simulink library "robolocks"  (Simulink 7.6)
settings: Solver=ode45  StartTime=0.0  StopTime=10.0  RelTol=1e-3
values from neighbouring files (symbols this model uses):
  q = 1    [quadrotor_plot.m]
  z = x(1:3)    [nrotor_dynamics.m]    (also in quadrotor_dynamics.m; quadrotor_plot.m = [u(1);u(2);u(3)])
undefined symbols (not defined in the file or in its folder): angdiff, Bicycle, cam, camera, camera2, Circle, cond, delta2tr, Dynamics, eul2T, eul2tr, fkine, ijacob, Inverse, invJac, jacob0, jacobn, jtraj, lspb, numcols, pinvJac, Plot, points, qd, qdd, Quadcopter, RNE, rne, roblocks_old, robot, Robot, rpy2T, rpy2tr, T2eul, T2rpy, T2xyz, test, tr2delta, tr2diff, tr2eul, tr2rpy, transl, trnorm, trotx, xyz2T
settings Model: Creator=n6334687  LastModifiedBy=n6334687

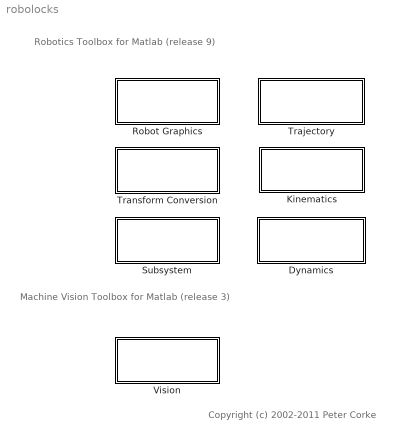
== system robolocks ==
  note: Robotics Toolbox for Matlab
      | (release 9)
  note: Machine Vision Toolbox for Matlab
      | (release 3)
  note: Copyright (c) 2002-2011 Peter Corke
  Dynamics : Subsystem
      mask Display:
      | color('darkBlue')
      | disp('Dynamics')
  Kinematics : Subsystem  AncestorBlock=test/Dynamics
      mask Display:
      | color('darkBlue')
      | disp('Kinematics')
  Robot Graphics : Subsystem  AncestorBlock=test/Plot
      mask Display:
      | color('darkBlue')
      | disp('Robot Graphics')
  Subsystem : Subsystem
      mask Display:
      | color('darkBlue')
      | disp('Transform')
  "Trajectory " : Subsystem
      mask Display:
      | color('darkBlue')
      | disp('Trajectory')
  Transform Conversion : Subsystem
      mask Display:
      | color('darkBlue')
      | disp('Transform Conversion')
  Vision : Subsystem
      mask Display:
      | color('Black')
      | disp('Vision')

== system robolocks/Dynamics ==
  note: Dynamics
  note: Arm-type robot
  note: Quadcopter
  note: Mobile robot
  Bicycle : Subsystem  AncestorBlock=roblocks_old/Bicycle  mask{accel=1, vlim=1, alim=2, x0=[0, 0, 0], handbrake=0}
      mask prompts: accel "Acceleration"; vlim "Velocity limit"; alim "Steering limits"; x0 "Initial state (x, y, theta)"
  Control Mixer : Subsystem  AncestorBlock=roblocks_old/Control Mixer
  Quadcopter : Subsystem  AncestorBlock=roblocks_old/Quadcopter  mask{quad=0}
      mask prompts: quad "Quadcopter params"
  RNE : Subsystem  AncestorBlock=roblocks_old/RNE  mask{robot=robot, grav=[0 0 9.81]}
      mask prompts: robot "Robot object"; grav "Gravity"
      mask help: Rigid-body inverse dynamics.
      mask init:
      | if isa(robot, 'SerialLink')
      |     n = robot.n
      |     rname = robot.name;
      | else
      |     n = 0;
      |     rname = '';
      | end
      mask Help: Given a robot dynamic model and joint angle, rate and acceleration determine the required joint torque.  Useful for computed and inverse torque control schemes.
      mask Display:
      | port_label('output', 1, 'Q')
      | port_label('input', 1, 'q')
      | port_label('input', 2, 'qd')
      | port_label('input', 3, 'qdd')
      | text(0.9, 0.9,  rname, 'horizontalAlignment', 'right')
  Robot : Subsystem  AncestorBlock=roblocks_old/Robot  mask{robot=robot, q0=[0 0 0 0 0 0]}
      mask prompts: robot "Robot object"; q0 "Initial state"
      mask help: Rigid-body dynamic model of robot.
      mask init:
      | if isa(robot, 'SerialLink')
      |     rname = robot.name;
      |     fprintf('**robot name is %s\n', rname);
      | else
      |     rname = '';
      |     n = 0
      | end
      mask Help: Simulates the forward (direct) rigid-body dynamics of the robot described by the given robot object.
      mask Display:
      | port_label('input', 1, 'Q')
      | port_label('output', 1, 'q')
      | port_label('output', 2, 'qd')
      | port_label('output', 3, 'qdd')
      | text(0.1, 0.9,  rname, 'horizontalAlignment', 'left')
  wires:
  ? -> RNE/2(qd)

== system robolocks/Kinematics ==
  note: Kinematics
  fkine : Subsystem  AncestorBlock=roblocks_old/fkine  mask{robot=robot}
      mask prompts: robot "Robot object"
      mask help: Robot forward kinematics.
      mask Help: Compute homogeneous transform for robot end-effector given joint angles.
      mask Display:
      | port_label('input', 1, 'q')
      | port_label('output', 1, 'T')
      | text(0.9, 0.9, robot.name,  'horizontalAlignment', 'right')
  ijacob : Subsystem  AncestorBlock=roblocks_old/ijacob
      mask Description:
      | Robot inverse Jacobian for world coordinates.
      | 
      | Only valid for square jacobians (ie/ 6DOF robots)
      mask Display:
      | text(0.4, 0.7, 'J', 'verticalAlignment', 'top', 'horizontalAlignment', 'left')
      | text(0.65, 0.65, '-1', 'verticalAlignment', 'bottom', 'horizontalAlignment', 'right')
      | port_label('input', 1, 'J');
      | port_label('output', 1, 'Ji')
  "jacob0 " : Subsystem  AncestorBlock=roblocks_old/jacob0  mask{robot=robot}
      mask prompts: robot "Robot object"
      mask help: Robot Jacobian for end-effector coordinates
      mask init:
      | n=robot.n;
      mask Display:
      | text(0.4, 0.7, 'J', 'verticalAlignment', 'top', 'horizontalAlignment', 'left')
      | text(0.4, 0.7, '0', 'verticalAlignment', 'bottom', 'horizontalAlignment', 'right')
      | text(0.5, 0.2, robot.name,  'horizontalAlignment', 'center')
      | port_label('input', 1, 'q')
      | port_label('output', 1, 'J')
  jacobn : Subsystem  AncestorBlock=roblocks_old/jacobn  mask{robot=robot}
      mask prompts: robot "Robot object"
      mask help: Robot Jacobian for end-effector coordinates
      mask init:
      | n=robot.n;
      mask Display:
      | text(0.5, 0.4, 'J', 'verticalAlignment', 'top', 'horizontalAlignment', 'left')
      | text(0.5, 0.4, 'n', 'verticalAlignment', 'bottom', 'horizontalAlignment', 'right')
      | text(0.9, 0.9, robot.name,  'horizontalAlignment', 'right')
      | port_label('input', 1, 'q')
      | port_label('output', 1, 'J')
  tr2diff : Subsystem  AncestorBlock=roblocks_old/tr2diff  mask{robot=robot}
      mask prompts: robot "Robot object"
      mask help: Robot forward kinematics.
      mask Help: Compute homogeneous transform for robot end-effector given joint angles.
      mask Display:
      | port_label('input', 1, 'T1')
      | port_label('input', 2, 'T2')
      | port_label('output', 1, 'dx')

== system robolocks/Robot Graphics ==
  note: Robot
      | Graphics
  Quadcopter plot : Subsystem  AncestorBlock=roblocks_old/Quadcopter plot
  plot : Subsystem  AncestorBlock=roblocks_old/plot  mask{robot=robot}
      mask prompts: robot "Name of robot"
      mask help: Graphical robot display.
      mask init:
      | if isa(robot, 'SerialLink')
      |     plot(robot,zeros(1,robot.n));
      | rname = robot.name;
      | fprintf('**robot name is %s\n', rname);
      | else
      |     rname = '';
      | end
      mask Help: This block graphically displays the named robot
      mask Display:
      | text(0.5, 0.9,  rname, 'horizontalAlignment', 'center')
      | port_label('input', 1, 'q')

== system robolocks/Subsystem ==
  note: Transform
  Inverse : Subsystem  AncestorBlock=roblocks_old/Inverse
  Post multiply : Subsystem  AncestorBlock=roblocks_old/Post multiply  mask{T2=0}
      mask help: Premultiply incoming transform by a constant transformation
  Pre multiply : Subsystem  AncestorBlock=roblocks_old/Pre multiply  mask{T=0}
      mask prompts: T "T1"
      mask help: Post multiply incoming transform by constant transform.

== system robolocks/Trajectory  ==
  note: Trajectory
  Circle : Subsystem  AncestorBlock=roblocks_old/Circle  mask{radius=1, freq=0.2}
      mask prompts: freq "Frequency (rev/s)"
  angdiff : Subsystem  AncestorBlock=roblocks_old/angdiff
  jtraj : Subsystem  AncestorBlock=roblocks_old/jtraj  mask{q0=[0 0 0 0 0 0], qf=[pi/4 pi/2 -pi/2 0 0 0], tmax=10}
      mask help: Joint interpolated trajectory.
      mask init:
      | n = length(q0);
      | if length(q0) ~= length(qf) ,
      |  error('q0 and qf must be same length')
      | end
      | t=[0:100]'/100*tmax;
      | [q,qd,qdd] = jtraj(q0, qf, t);
      mask Help:
      | Generate quintic polynomial to move from initial to final joint angles as specified.  Initial and final velocity are assumed to be zero.
      | 
      | Outputs joint angles as well as joint angle rates.
      mask Display:
      | port_label('output', 1, 'q')
      | port_label('output', 2, 'qd')
      | port_label('output', 3, 'qdd')
  lspb : Subsystem  AncestorBlock=roblocks_old/lspb  mask{q0=0, qf=0, tmax=0}
      mask help: Scalar trajectory.
      mask init:
      | n = length(q0);
      | if length(q0) ~= length(qf) ,
      |  error('q0 and qf must be same length')
      | end
      | t=[0:1000]'/1000*tmax;
      | [q,qd,qdd] = lspb(q0, qf, t);
      mask Help:
      | Generate linear segment with polynomial blend to move from initial to final joint angles as specified.  Initial and final velocity are assumed to be zero.
      | 
      | Outputs joint angles as well as joint angle rates and acceleration.
  pose integral : Subsystem  AncestorBlock=roblocks_old/pose integral  mask{T0=transl(1,1,-3)*trotx(0.2), dt=0.02}
      mask prompts: T0 "Initial pose (hom transform)"; dt "Sample interval (s)"

== system robolocks/Transform Conversion ==
  note: Transform
      | conversion
  T2eul : Subsystem  AncestorBlock=roblocks_old/T2eul
      mask Description: Convert transform to Euler angles.
  T2rpy : Subsystem  AncestorBlock=roblocks_old/T2rpy
      mask Description: Convert transform to roll/pitch/yaw angles.
  T2xyz : Subsystem  AncestorBlock=roblocks_old/T2xyz
      mask Description: Convert transform to xyz scalars
  eul2T : Subsystem  AncestorBlock=roblocks_old/eul2T
      mask Description: Convert Euler angles to transform.
  rpy2T : Subsystem  AncestorBlock=roblocks_old/rpy2T
      mask Description: Convert roll/pitch/yaw angles to transform.
  xyz2T : Subsystem  AncestorBlock=roblocks_old/xyz2T
      mask Description: Convert xyz scalars to transform.

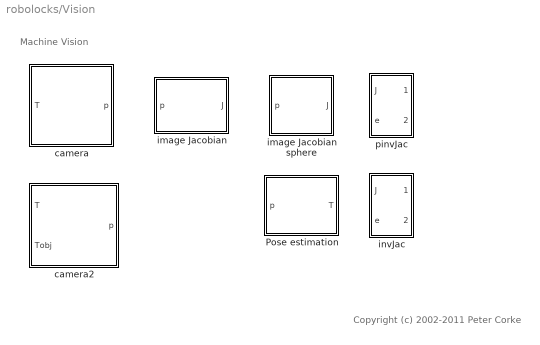
== system robolocks/Vision ==
  note: Machine Vision
  note: Copyright (c) 2002-2011 Peter Corke
  Pose estimation : Subsystem  AncestorBlock=roblocks_old/Pose estimation  mask{cam=0, P=0}
      mask prompts: cam "Camera"; P "Points (3xN)"
  camera : Subsystem  AncestorBlock=roblocks_old/camera  mask{cam=, points=}
      mask prompts: cam "Camera"; points "Points (3xN)"
  camera2 : Subsystem  AncestorBlock=roblocks_old/camera2
  image Jacobian : Subsystem  AncestorBlock=roblocks_old/image Jacobian  mask{cam=, z=}
      mask prompts: cam "Camera"; z "Assumed depth (m)"
  image Jacobian sphere : Subsystem  AncestorBlock=|
      | roblocks_old/image
      | Jacobian
      | sphere
  invJac : Subsystem  AncestorBlock=roblocks_old/invJac
  pinvJac : Subsystem  AncestorBlock=roblocks_old/pinvJac

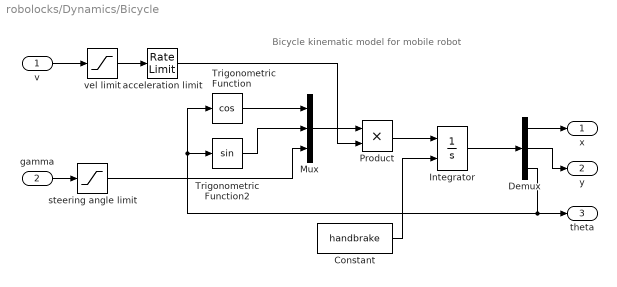
== system robolocks/Dynamics/Bicycle ==
  note: Bicycle kinematic model for mobile robot
  v : Inport
  gamma : Inport  Port=2
  Constant : Constant  Value=handbrake
  Demux : Demux  Outputs=3
  Integrator : Integrator  ExternalReset=level  InitialCondition=x0
  Mux : Mux  Inputs=3
  Product : Product  RndMeth=Zero
  Trigonometric Function : Trigonometry  Operator=cos
  Trigonometric Function2 : Trigonometry
  acceleration limit : RateLimiter  RisingSlewLimit=accel  FallingSlewLimit=-accel  SampleTimeMode=inherited
  steering angle limit : Saturate  UpperLimit=alim  LowerLimit=-alim
  vel limit : Saturate  UpperLimit=vlim  LowerLimit=-vlim
  x : Outport
  y : Outport  Port=2
  theta : Outport  Port=3
  wires:
  Constant/1 -> Integrator/2
  steering angle limit/1 -> Mux/3
  Trigonometric Function2/1 -> Mux/2
  vel limit/1 -> acceleration limit/1
  Mux/1 -> Product/1
  v/1 -> vel limit/1
  gamma/1 -> steering angle limit/1
  Demux/2 -> y/1
  Demux/1 -> x/1
  Demux/3 -> theta/1, Trigonometric Function2/1, Trigonometric Function/1
  Integrator/1 -> Demux/1
  Product/1 -> Integrator/1
  acceleration limit/1 -> Product/2
  Trigonometric Function/1 -> Mux/1

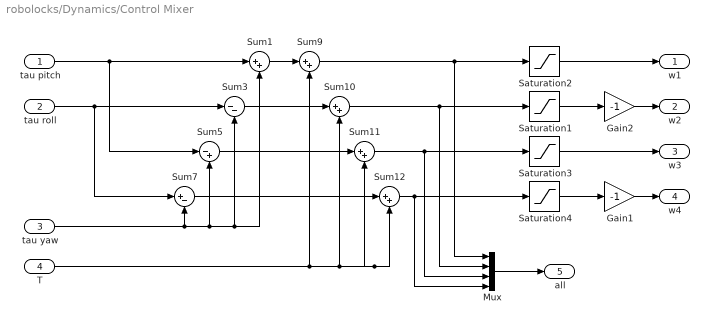
== system robolocks/Dynamics/Control Mixer ==
  tau pitch : Inport
  tau roll : Inport  Port=2
  tau yaw : Inport  Port=3
  T : Inport  Port=4
  Gain1 : Gain  Gain=-1
  Gain2 : Gain  Gain=-1
  Mux : Mux
  Saturation{1..4} (4 alike) : Saturate  UpperLimit=1000  LowerLimit=700
  Sum{1,9..12} (5 alike) : Sum  Inputs=|++  SaturateOnIntegerOverflow=on  InputSameDT=on  OutDataTypeStr=Inherit: Same as first input
  Sum3 : Sum  Inputs=|--  SaturateOnIntegerOverflow=on  InputSameDT=on  OutDataTypeStr=Inherit: Same as first input
  Sum5 : Sum  Inputs=|-+  SaturateOnIntegerOverflow=on  InputSameDT=on  OutDataTypeStr=Inherit: Same as first input
  Sum7 : Sum  Inputs=|+-  SaturateOnIntegerOverflow=on  InputSameDT=on  OutDataTypeStr=Inherit: Same as first input
  w1 : Outport
  w2 : Outport  Port=2
  w3 : Outport  Port=3
  w4 : Outport  Port=4
  all : Outport  Port=5
  wires:
  Gain1/1 -> w4/1
  Gain2/1 -> w2/1
  Mux/1 -> all/1
  tau roll/1 -> Sum7/1, Sum3/1
  T/1 -> Sum9/2, Sum10/2, Sum11/2, Sum12/2
  Sum12/1 -> Mux/4, Saturation4/1
  Sum11/1 -> Mux/3, Saturation3/1
  Sum10/1 -> Mux/2, Saturation1/1
  Sum9/1 -> Mux/1, Saturation2/1
  Sum7/1 -> Sum12/1
  Sum5/1 -> Sum11/1
  Sum3/1 -> Sum10/1
  Sum1/1 -> Sum9/1
  tau pitch/1 -> Sum5/1, Sum1/1
  Saturation4/1 -> Gain1/1
  Saturation3/1 -> w3/1
  Saturation1/1 -> Gain2/1
  Saturation2/1 -> w1/1
  tau yaw/1 -> Sum1/2, Sum3/2, Sum5/2, Sum7/2

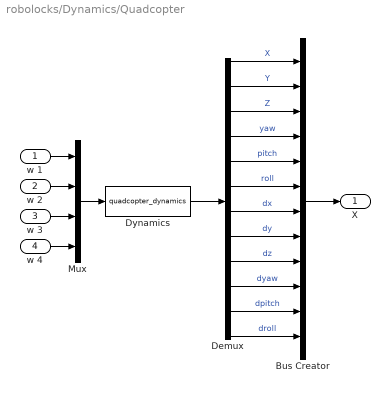
== system robolocks/Dynamics/Quadcopter ==
  w 1 : Inport
  w 2 : Inport  Port=2
  w 3 : Inport  Port=3
  w 4 : Inport  Port=4
  Bus Creator : BusCreator  Inputs='X','Y','Z','yaw','pitch','roll','dx','dy','dz','dyaw','dpitch','droll'
  Demux : Demux  Outputs=12
  Dynamics : S-Function  FunctionName=quadcopter_dynamics  Parameters=quad  EnableBusSupport=off
  Mux : Mux
  X : Outport
  wires:
  Demux/12 -> Bus Creator/12  "droll"
  Demux/11 -> Bus Creator/11  "dpitch"
  Demux/10 -> Bus Creator/10  "dyaw"
  Dynamics/1 -> Demux/1
  Bus Creator/1 -> X/1
  Demux/8 -> Bus Creator/8  "dy"
  Demux/6 -> Bus Creator/6  "roll"
  Demux/2 -> Bus Creator/2  "Y"
  Demux/9 -> Bus Creator/9  "dz"
  Demux/7 -> Bus Creator/7  "dx"
  w 4/1 -> Mux/4
  w 3/1 -> Mux/3
  w 2/1 -> Mux/2
  w 1/1 -> Mux/1
  Demux/5 -> Bus Creator/5  "pitch"
  Demux/4 -> Bus Creator/4  "yaw"
  Demux/3 -> Bus Creator/3  "Z"
  Demux/1 -> Bus Creator/1  "X"
  Mux/1 -> Dynamics/1

== system robolocks/Dynamics/RNE ==
  q : Inport
  qd : Inport  Port=2
  qdd : Inport  Port=3
  MATLAB Fcn : MATLABFcn  MATLABFcn=rne(robot, u(1:n)', u(n+1:2*n)', u(2*n+1:3*n)')  OutputDimensions=n
  Mux : Mux  Inputs=3
  Q : Outport
  wires:
  Mux/1 -> MATLAB Fcn/1
  q/1 -> Mux/1
  qd/1 -> Mux/2
  qdd/1 -> Mux/3
  MATLAB Fcn/1 -> Q/1

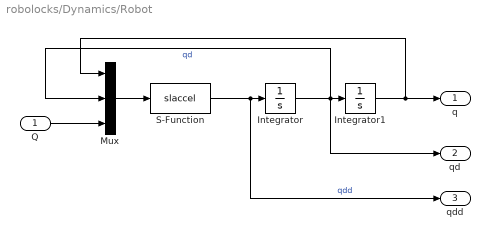
== system robolocks/Dynamics/Robot ==
  Q : Inport
  Integrator : Integrator
  Integrator1 : Integrator
  Mux : Mux  Inputs=3
  S-Function : S-Function  FunctionName=slaccel  Parameters=robot  EnableBusSupport=off
  q : Outport
  qd : Outport  Port=2
  qdd : Outport  Port=3
  wires:
  Integrator1/1 -> Mux/1, q/1
  Q/1 -> Mux/3
  Integrator/1 -> Mux/2, Integrator1/1, qd/1  "qd"
  Mux/1 -> S-Function/1
  S-Function/1 -> Integrator/1, qdd/1  "qdd"

== system robolocks/Kinematics/fkine ==
  q : Inport
  MATLAB Fcn : MATLABFcn  MATLABFcn=fkine(robot,u)  OutputDimensions=[4 4]  Output1D=off
  T : Outport
  wires:
  MATLAB Fcn/1 -> T/1
  q/1 -> MATLAB Fcn/1

== system robolocks/Kinematics/ijacob ==
  J : Inport
  inverse jacobian : MATLABFcn  MATLABFcn=inv(u)  Output1D=off
  Ji : Outport
  wires:
  J/1 -> inverse jacobian/1
  inverse jacobian/1 -> Ji/1

== system robolocks/Kinematics/jacob0  ==
  q : Inport
  MATLAB Fcn : MATLABFcn  MATLABFcn=jacob0(robot,u)  OutputDimensions=[6 n]  Output1D=off
  J : Outport
  wires:
  q/1 -> MATLAB Fcn/1
  MATLAB Fcn/1 -> J/1

== system robolocks/Kinematics/jacobn ==
  q : Inport
  MATLAB Fcn : MATLABFcn  MATLABFcn=jacobn(robot,u)  OutputDimensions=[6 n]  Output1D=off
  J : Outport
  wires:
  q/1 -> MATLAB Fcn/1
  MATLAB Fcn/1 -> J/1

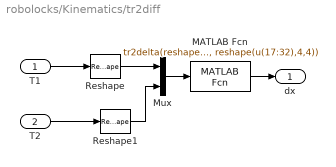
== system robolocks/Kinematics/tr2diff ==
  T1 : Inport
  T2 : Inport  Port=2
  MATLAB Fcn : MATLABFcn  MATLABFcn=tr2delta(reshape(u(1:16),4,4), reshape(u(17:32),4,4))  OutputDimensions=6
  Mux : Mux  Inputs=2
  Reshape : Reshape
  Reshape1 : Reshape
  dx : Outport
  wires:
  Reshape1/1 -> Mux/2
  Reshape/1 -> Mux/1
  Mux/1 -> MATLAB Fcn/1
  T2/1 -> Reshape1/1
  T1/1 -> Reshape/1
  MATLAB Fcn/1 -> dx/1

== system robolocks/Robot Graphics/Quadcopter plot ==
  X : Inport
  Bus Selector1 : BusSelector  OutputSignals=X,Y,Z,yaw,pitch,roll  OutputAsBus=on
  Plotter : S-Function  FunctionName=quadcopter_plot  Parameters=[2,10], 1, 1  EnableBusSupport=off
  wires:
  Bus Selector1/1 -> Plotter/1
  X/1 -> Bus Selector1/1

== system robolocks/Robot Graphics/plot ==
  q : Inport
  S-Function : S-Function  FunctionName=slplotbot  Parameters=robot  EnableBusSupport=off
  wires:
  q/1 -> S-Function/1

== system robolocks/Subsystem/Inverse ==
  T : Inport
  MATLAB Fcn : MATLABFcn  MATLABFcn=inv(u)  OutputDimensions=[4,4]  Output1D=off
  invT : Outport
  wires:
  MATLAB Fcn/1 -> invT/1
  T/1 -> MATLAB Fcn/1

== system robolocks/Subsystem/Post multiply ==
  T1 : Inport
  Constant : Constant  Value=T2
  Product : Product  Multiplication=Matrix(*)  RndMeth=Zero
  T : Outport
  wires:
  T1/1 -> Product/1
  Constant/1 -> Product/2
  Product/1 -> T/1

== system robolocks/Subsystem/Pre multiply ==
  T2 : Inport
  Constant : Constant  Value=T  VectorParams1D=off
  Product : Product  Multiplication=Matrix(*)  RndMeth=Zero
  T : Outport
  wires:
  T2/1 -> Product/2
  Product/1 -> T/1
  Constant/1 -> Product/1

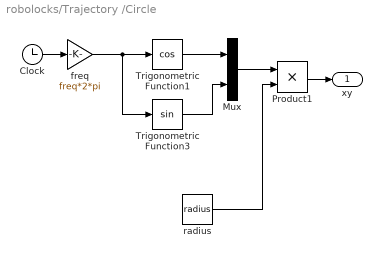
== system robolocks/Trajectory /Circle ==
  Clock : Clock
      settings: Decimation=10
  Mux : Mux  Inputs=2
  Product1 : Product  RndMeth=Zero
  Trigonometric Function1 : Trigonometry  Operator=cos
  Trigonometric Function3 : Trigonometry
  freq : Gain  Gain=freq*2*pi
  radius : Constant  Value=radius
  xy : Outport
  wires:
  Trigonometric Function3/1 -> Mux/2
  Trigonometric Function1/1 -> Mux/1
  Mux/1 -> Product1/1
  radius/1 -> Product1/2
  Clock/1 -> freq/1
  Product1/1 -> xy/1
  freq/1 -> Trigonometric Function1/1, Trigonometric Function3/1

== system robolocks/Trajectory /angdiff ==
  + : Inport
  - : Inport  Port=2
  MATLAB Fcn : MATLABFcn  MATLABFcn=angdiff(u(1), u(2))
  Mux : Mux  Inputs=2
  d : Outport
  wires:
  -/1 -> Mux/2
  MATLAB Fcn/1 -> d/1
  Mux/1 -> MATLAB Fcn/1
  +/1 -> Mux/1

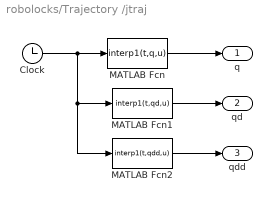
== system robolocks/Trajectory /jtraj ==
  Clock : Clock
      settings: Decimation=10
  MATLAB Fcn : MATLABFcn  MATLABFcn=interp1(t,q,u)  OutputDimensions=n
  MATLAB Fcn1 : MATLABFcn  MATLABFcn=interp1(t,qd,u)  OutputDimensions=n
  MATLAB Fcn2 : MATLABFcn  MATLABFcn=interp1(t,qdd,u)  OutputDimensions=n
  q : Outport
  qd : Outport  Port=2
  qdd : Outport  Port=3
  wires:
  MATLAB Fcn2/1 -> qdd/1
  Clock/1 -> MATLAB Fcn2/1, MATLAB Fcn1/1, MATLAB Fcn/1
  MATLAB Fcn1/1 -> qd/1
  MATLAB Fcn/1 -> q/1

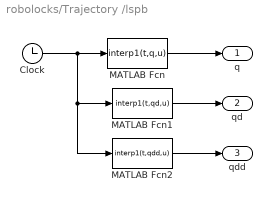
== system robolocks/Trajectory /lspb ==
  Clock : Clock
      settings: Decimation=10
  MATLAB Fcn : MATLABFcn  MATLABFcn=interp1(t,q,u)  OutputDimensions=n
  MATLAB Fcn1 : MATLABFcn  MATLABFcn=interp1(t,qd,u)  OutputDimensions=n
  MATLAB Fcn2 : MATLABFcn  MATLABFcn=interp1(t,qdd,u)  OutputDimensions=n
  q : Outport
  qd : Outport  Port=2
  qdd : Outport  Port=3
  wires:
  MATLAB Fcn/1 -> q/1
  MATLAB Fcn1/1 -> qd/1
  Clock/1 -> MATLAB Fcn/1, MATLAB Fcn1/1, MATLAB Fcn2/1
  MATLAB Fcn2/1 -> qdd/1

== system robolocks/Trajectory /pose integral ==
  v : Inport
  MATLAB Fcn3 : MATLABFcn  MATLABFcn=delta2tr(u)  Output1D=off
  Product : Product  Multiplication=Matrix(*)  RndMeth=Zero
  Unit Delay : UnitDelay  X0=T0  SampleTime=dt
  trnorm : MATLABFcn  MATLABFcn=trnorm(u)  Output1D=off
  T : Outport
  wires:
  v/1 -> MATLAB Fcn3/1
  trnorm/1 -> Unit Delay/1
  MATLAB Fcn3/1 -> Product/1
  Unit Delay/1 -> T/1, Product/2
  Product/1 -> trnorm/1

== system robolocks/Transform Conversion/T2eul ==
  T : Inport
  Demux : Demux  Outputs=3
  MATLAB Fcn : MATLABFcn  MATLABFcn=tr2eul(u)  OutputDimensions=3
  a : Outport
  b : Outport  Port=2
  c : Outport  Port=3
  wires:
  T/1 -> MATLAB Fcn/1
  MATLAB Fcn/1 -> Demux/1
  Demux/1 -> a/1
  Demux/2 -> b/1
  Demux/3 -> c/1

== system robolocks/Transform Conversion/T2rpy ==
  T : Inport
  Demux : Demux  Outputs=3
  MATLAB Fcn : MATLABFcn  MATLABFcn=tr2rpy(u)  OutputDimensions=3
  roll : Outport
  pitch : Outport  Port=2
  yaw : Outport  Port=3
  wires:
  T/1 -> MATLAB Fcn/1
  MATLAB Fcn/1 -> Demux/1
  Demux/1 -> roll/1
  Demux/2 -> pitch/1
  Demux/3 -> yaw/1

== system robolocks/Transform Conversion/T2xyz ==
  T : Inport
  Demux : Demux  Outputs=3
  MATLAB Fcn : MATLABFcn  MATLABFcn=transl(u)  OutputDimensions=3
  x : Outport
  y : Outport  Port=2
  z : Outport  Port=3
  wires:
  Demux/3 -> z/1
  Demux/2 -> y/1
  Demux/1 -> x/1
  MATLAB Fcn/1 -> Demux/1
  T/1 -> MATLAB Fcn/1

== system robolocks/Transform Conversion/eul2T ==
  a : Inport
  b : Inport  Port=2
  c : Inport  Port=3
  MATLAB Fcn : MATLABFcn  MATLABFcn=eul2tr(u)  OutputDimensions=[4 4]  Output1D=off
  Mux : Mux  Inputs=3
  T : Outport
  wires:
  b/1 -> Mux/2
  a/1 -> Mux/1
  Mux/1 -> MATLAB Fcn/1
  MATLAB Fcn/1 -> T/1
  c/1 -> Mux/3

== system robolocks/Transform Conversion/rpy2T ==
  roll : Inport
  pitch : Inport  Port=2
  yaw : Inport  Port=3
  MATLAB Fcn : MATLABFcn  MATLABFcn=rpy2tr(u)  OutputDimensions=[4 4]  Output1D=off
  Mux : Mux  Inputs=3
  T : Outport
  wires:
  pitch/1 -> Mux/2
  roll/1 -> Mux/1
  Mux/1 -> MATLAB Fcn/1
  MATLAB Fcn/1 -> T/1
  yaw/1 -> Mux/3

== system robolocks/Transform Conversion/xyz2T ==
  x : Inport
  y : Inport  Port=2
  z : Inport  Port=3
  MATLAB Fcn : MATLABFcn  MATLABFcn=transl(u)  OutputDimensions=[4 4]  Output1D=off
  Mux : Mux  Inputs=3
  T : Outport
  wires:
  z/1 -> Mux/3
  MATLAB Fcn/1 -> T/1
  Mux/1 -> MATLAB Fcn/1
  x/1 -> Mux/1
  y/1 -> Mux/2

== system robolocks/Vision/Pose estimation ==
  p : Inport
  MATLAB Fcn : MATLABFcn  MATLABFcn=cam.estpose(P, u)  OutputDimensions=[4,4]  Output1D=off
  T : Outport
  wires:
  MATLAB Fcn/1 -> T/1
  p/1 -> MATLAB Fcn/1

== system robolocks/Vision/camera ==
  T : Inport
  MATLAB Fcn : MATLABFcn  MATLABFcn=cam.plot(points, 'Tcam', u, 'drawnow')  OutputDimensions=[2,numcols(points)]  OutputSignalType=real  Output1D=off
  p : Outport
  wires:
  T/1 -> MATLAB Fcn/1
  MATLAB Fcn/1 -> p/1

== system robolocks/Vision/camera2 ==
  T : Inport
  Tobj : Inport  Port=2
  MATLAB Fcn : MATLABFcn  MATLABFcn=cam.plot(points, 'Tcam', u(:,:,1), 'Tobj', u(:,:,2), 'drawnow')  OutputDimensions=[2,numcols(points)]  OutputSignalType=real  Output1D=off
  Matrix Concatenate : Concatenate  Mode=Multidimensional array  ConcatenateDimension=3
  p : Outport
  wires:
  T/1 -> Matrix Concatenate/1
  Tobj/1 -> Matrix Concatenate/2
  Matrix Concatenate/1 -> MATLAB Fcn/1
  MATLAB Fcn/1 -> p/1

== system robolocks/Vision/image Jacobian ==
  p : Inport
  MATLAB Fcn : MATLABFcn  MATLABFcn=cam.visjac_p(u, z)  Output1D=off
  J : Outport
  wires:
  p/1 -> MATLAB Fcn/1
  MATLAB Fcn/1 -> J/1

== system robolocks/Vision/image Jacobian sphere ==
  p : Inport
  MATLAB Fcn : MATLABFcn  MATLABFcn=cam.visjac_p(u, z)  Output1D=off
  J : Outport
  wires:
  p/1 -> MATLAB Fcn/1
  MATLAB Fcn/1 -> J/1

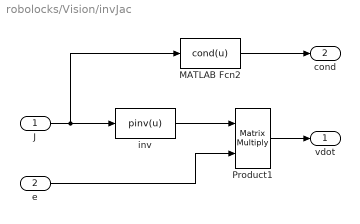
== system robolocks/Vision/invJac ==
  J : Inport
  e : Inport  Port=2
  MATLAB Fcn2 : MATLABFcn  MATLABFcn=cond(u)  Output1D=off
  Product1 : Product  Multiplication=Matrix(*)  SaturateOnIntegerOverflow=on  RndMeth=Zero  InputSameDT=on  OutDataTypeStr=Inherit: Same as first input
  inv : MATLABFcn  MATLABFcn=pinv(u)  Output1D=off
  vdot : Outport
  cond : Outport  Port=2
  wires:
  Product1/1 -> vdot/1
  MATLAB Fcn2/1 -> cond/1
  e/1 -> Product1/2
  inv/1 -> Product1/1
  J/1 -> inv/1, MATLAB Fcn2/1

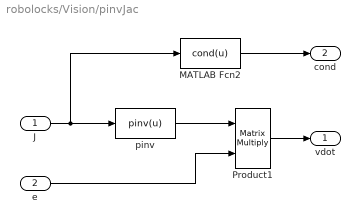
== system robolocks/Vision/pinvJac ==
  J : Inport
  e : Inport  Port=2
  MATLAB Fcn2 : MATLABFcn  MATLABFcn=cond(u)  Output1D=off
  Product1 : Product  Multiplication=Matrix(*)  SaturateOnIntegerOverflow=on  RndMeth=Zero  InputSameDT=on  OutDataTypeStr=Inherit: Same as first input
  pinv : MATLABFcn  MATLABFcn=pinv(u)  Output1D=off
  vdot : Outport
  cond : Outport  Port=2
  wires:
  Product1/1 -> vdot/1
  MATLAB Fcn2/1 -> cond/1
  e/1 -> Product1/2
  pinv/1 -> Product1/1
  J/1 -> pinv/1, MATLAB Fcn2/1
